simulink model "Isim"  (R2020a)
settings: Solver=VariableStepAuto  StartTime=0.0  StopTime=100  MaxStep=1e-2  RelTol=1e-3
values from neighbouring files (symbols this model uses):
  I0 = 2    [ErroQuadratico.m]    (also in ErroQuadraticoSIR.m)
  S0 = 60e6    (= 60000000)    [ErroQuadratico.m]    (also in ErroQuadraticoSIR.m)
undefined symbols (not defined in the file or in its folder): beta0, r0
settings Model: Creator=a1  LastModifiedBy=a1

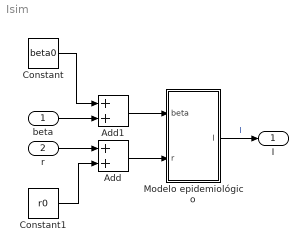
== system Isim ==
  beta : Inport
  r : Inport  Port=2
  Add : Sum
  Add1 : Sum
  Constant : Constant  Value=beta0
  Constant1 : Constant  Value=r0
  Modelo epidemiológico : Subsystem
  I : Outport
  wires:
  Modelo epidemiológico/1(I) -> I/1  "I"
  r/1 -> Add/1
  beta/1 -> Add1/2
  Add/1 -> Modelo epidemiológico/2(r)
  Constant/1 -> Add1/1
  Constant1/1 -> Add/2
  Add1/1 -> Modelo epidemiológico/1(beta)

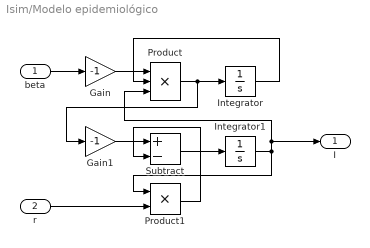
== system Isim/Modelo epidemiológico ==
  beta : Inport
  r : Inport  Port=2
  Gain : Gain  Gain=-1
  Gain1 : Gain  Gain=-1
  Integrator : Integrator  InitialCondition=S0
  Integrator1 : Integrator  InitialCondition=I0
  Product : Product  Inputs=3
  Product1 : Product
  Subtract : Sum  Inputs=+-
  I : Outport
  wires:
  beta/1 -> Gain/1
  Gain1/1 -> Subtract/1
  Gain/1 -> Product/1
  Product1/1 -> Subtract/2
  Subtract/1 -> Integrator1/1
  Product/1 -> Gain1/1, Integrator/1
  r/1 -> Product1/2
  Integrator/1 -> Product/2
  Integrator1/1 -> Product1/1, I/1, Product/3
